simulink model "A20220204b_ES1_sim"  (R2022b)
settings: Solver=VariableStepAuto  StartTime=0.0  StopTime=10.0  RelTol=1e-3
settings Model: Creator=claudio  LastModifiedBy=claudio

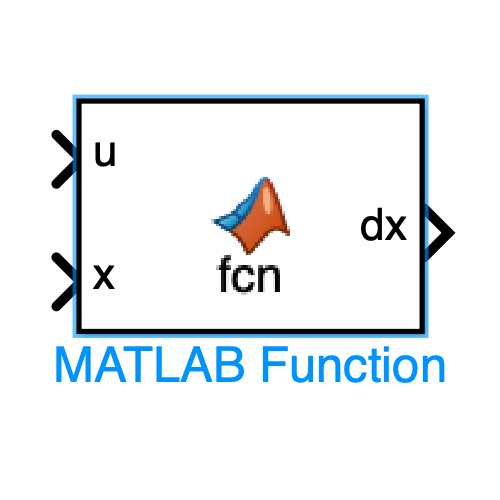
[thumbnail: Simulink's stored preview of the top-level diagram]
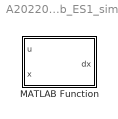
== system A20220204b_ES1_sim ==
  MATLAB Function : MATLAB Function  TreatAsAtomicUnit=on

== matlab function A20220204b_ES1_sim/MATLAB Function ==
  data: u input; dx output; x input
function dx = fcn(u,x)
x1=x(1);
x2=x(2);
dx=[x1*(0.01*x1-1)+(x1*x2)/50;0.001*x1*x2/1000-0.1*x2+u];
